simulink model "Microgrid_24h_Bhutan"  (Simulink 8.1)
settings: Solver=ode45  StartTime=0.0  StopTime=1  RelTol=1e-3
undefined symbols (not defined in the file or in its folder): Acid, Lead
libraries: powerlib x60, powerlib_extras x51, simulink x3, electricdrivelib x1
(part 2 of 2)

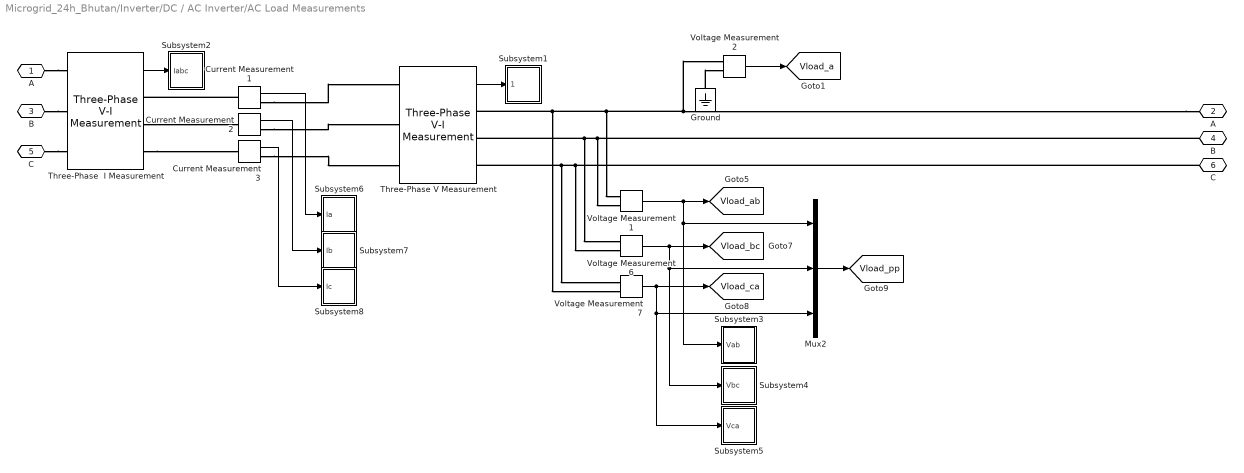
== system Microgrid_24h_Bhutan/Inverter/DC / AC Inverter/AC Load Measurements ==
  Current Measurement1 : powerlib/Measurements/Current Measurement  PhasorSimulation=off  OutputType=Complex  PSBequivalent=0
  Current Measurement2 : powerlib/Measurements/Current Measurement  PhasorSimulation=off  OutputType=Complex  PSBequivalent=0
  Current Measurement3 : powerlib/Measurements/Current Measurement  PhasorSimulation=off  OutputType=Complex  PSBequivalent=0
  Ground : powerlib/Elements/Ground  LConnTagsString=a
  Mux2 : Mux  Inputs=3
  Subsystem1 : Subsystem
  Subsystem2 : Subsystem
  Subsystem3 : Subsystem
  Subsystem4 : Subsystem
  Subsystem5 : Subsystem
  Subsystem6 : Subsystem
  Subsystem7 : Subsystem
  Subsystem8 : Subsystem
  Three-Phase V Measurement : powerlib/Measurements/Three-Phase V-I Measurement  VoltageMeasurement=phase-to-ground  SetLabelV=off  LabelV=Vabc  Vpu=off  VpuLL=off  CurrentMeasurement=no  SetLabelI=off  LabelI=Iabc  Ipu=off  Pbase=100e6  Vbase=500e3  OutputType=Complex  PhasorSimulation=off  PSBequivalent=0
  Three-Phase  I Measurement : powerlib/Measurements/Three-Phase V-I Measurement  VoltageMeasurement=no  SetLabelV=off  LabelV=Vabc  Vpu=off  VpuLL=off  CurrentMeasurement=yes  SetLabelI=off  LabelI=Iabc  Ipu=off  Pbase=100e6  Vbase=500e3  OutputType=Complex  PhasorSimulation=off  PSBequivalent=0
  Voltage Measurement{1..2,6..7} (4 alike) : powerlib/Measurements/Voltage Measurement  PhasorSimulation=off  OutputType=Complex  PSBequivalent=0
  A : PMIOPort  Port=1  Side=Left
  "A " : PMIOPort  Port=2  Side=Right
  B : PMIOPort  Port=3  Side=Left
  "B " : PMIOPort  Port=4  Side=Right
  C : PMIOPort  Port=5  Side=Left
  "C " : PMIOPort  Port=6  Side=Right
  tag scope: Vload_a=global, Vload_ab=global, Vload_bc=global, Vload_ca=global, Vload_pp=global
  wires:
  Three-Phase  I Measurement/1 -> Subsystem2/1(Iabc)
  Voltage Measurement1/1 -> [Vload_ab], Mux2/1, Subsystem3/1(Vab)
  Voltage Measurement6/1 -> [Vload_bc], Mux2/2, Subsystem4/1(Vbc)
  Voltage Measurement7/1 -> [Vload_ca], Mux2/3, Subsystem5/1(Vca)
  Mux2/1 -> [Vload_pp]
  Three-Phase V Measurement/1 -> Subsystem1/1(Vabc)
  Voltage Measurement2/1 -> [Vload_a]
  Current Measurement3/1 -> Subsystem8/1(Ic)
  Current Measurement2/1 -> Subsystem7/1(Ib)
  Current Measurement1/1 -> Subsystem6/1(Ia)
  connections:
  A/RConn1 -- Three-Phase  I Measurement/LConn1
  "A "/RConn1 -- Voltage Measurement1/LConn1 -- Three-Phase V Measurement/RConn1 -- Voltage Measurement7/LConn2 -- Voltage Measurement2/LConn1
  B/RConn1 -- Three-Phase  I Measurement/LConn2
  "B "/RConn1 -- Voltage Measurement1/LConn2 -- Three-Phase V Measurement/RConn2 -- Voltage Measurement6/LConn1
  C/RConn1 -- Three-Phase  I Measurement/LConn3
  "C "/RConn1 -- Voltage Measurement6/LConn2 -- Three-Phase V Measurement/RConn3 -- Voltage Measurement7/LConn1
  Ground/LConn1 -- Voltage Measurement2/LConn2
  Current Measurement1/LConn1 -- Three-Phase  I Measurement/RConn1
  Three-Phase  I Measurement/RConn2 -- Current Measurement2/LConn1
  Three-Phase  I Measurement/RConn3 -- Current Measurement3/LConn1
  Current Measurement3/RConn1 -- Three-Phase V Measurement/LConn3
  Current Measurement2/RConn1 -- Three-Phase V Measurement/LConn2
  Current Measurement1/RConn1 -- Three-Phase V Measurement/LConn1

== system Microgrid_24h_Bhutan/Inverter/DC BUS /Subsystem1 ==
  Idcinv : Inport
  LPF vq11 : powerlib_extras/Discrete  Control Blocks/Discrete 1st-Order Filter  FilterType=Lowpass  Tc=10e-3  Ts=5e-6  Initialize=off  Vac_Init=[0.8 -25 60]  Vdc_Init=0  PlotResponse=off  param1=[1 100 0.1]
  To Workspace1 : ToWorkspace  VariableName=Idcinv  SampleTime=-1
  To Workspace2 : ToWorkspace  VariableName=Idcinv1  SampleTime=-1
  tag scope: Idcinv=global
  wires:
  Idcinv/1 -> [Idcinv], To Workspace1/1, LPF vq11/1
  LPF vq11/1 -> To Workspace2/1

== system Microgrid_24h_Bhutan/Inverter/DC BUS /Subsystem2 ==
  Vdcinv : Inport
  LPF vq11 : powerlib_extras/Discrete  Control Blocks/Discrete 1st-Order Filter  FilterType=Lowpass  Tc=10e-3  Ts=5e-6  Initialize=off  Vac_Init=[0.8 -25 60]  Vdc_Init=0  PlotResponse=off  param1=[1 100 0.1]
  To Workspace1 : ToWorkspace  VariableName=Vdcinv  SampleTime=-1
  To Workspace2 : ToWorkspace  VariableName=Vdcinv1  SampleTime=-1
  tag scope: Vdcinv=global
  wires:
  Vdcinv/1 -> [Vdcinv], To Workspace1/1, LPF vq11/1
  LPF vq11/1 -> To Workspace2/1

== system Microgrid_24h_Bhutan/Inverter/Inverter Control/ Voltage Reference Generator ==
  Mux4 : Mux  Inputs=3
  Phase A reference : Sin  Amplitude=400*sqrt(2)/sqrt(3)  Frequency=2*pi*50  SampleTime=0
  Phase B reference : Sin  Amplitude=400*sqrt(2)/sqrt(3)  Frequency=2*pi*50  Phase=-2*pi/3  SampleTime=0
  Phase C reference : Sin  Amplitude=400*sqrt(2)/sqrt(3)  Frequency=2*pi*50  Phase=2*pi/3  SampleTime=0
  Product : Product  RndMeth=Zero
  Ramp : simulink/Sources/Ramp  slope=1/0.3  start=0  X0=0
  Saturation : Saturate  UpperLimit=1  LowerLimit=0
  Vabc* : Outport
  tag scope: Vabc_ref=global
  wires:
  Phase B reference/1 -> Mux4/2
  Phase A reference/1 -> Mux4/1
  Phase C reference/1 -> Mux4/3
  Ramp/1 -> Saturation/1
  Saturation/1 -> Product/2
  Mux4/1 -> Vabc*/1, [Vabc_ref]

== system Microgrid_24h_Bhutan/Inverter/Inverter Control/Cross Terms ==
  id* : Inport
  iq* : Inport  Port=2
  Gain1 : Gain  Gain=-2*pi*50*3e-3
  Gain2 : Gain  Gain=2*pi*50*3e-3
  " q" : Outport
  " d" : Outport  Port=2
  wires:
  id*/1 -> Gain1/1
  iq*/1 -> Gain2/1
  Gain1/1 -> " d"/1
  Gain2/1 -> " q"/1

== system Microgrid_24h_Bhutan/Inverter/Inverter Control/Current Ref. Generator ==
  note: evd
  note: evq
  evd : Inport
  evq : Inport  Port=2
  Divide : Product  Inputs=*/
  Divide1 : Product  Inputs=/*
  Scope24 : Scope
      settings: TimeRange=0.09  YMin=0.699626  YMax=0.699626  SaveName=ScopeData53
  Sum1 : Sum  Inputs=-+|
  Sum3 : Sum  Inputs=|++
  Zd : Gain  Gain=0.4559
  Zd1 : Gain  Gain=0.4559
  Zd^2+Zq^2 : Constant  Value=0.4559^2+0.1824^2
  Zq : Gain  Gain=0.1824
  Zq1 : Gain  Gain=0.1824
  id* : Outport
  iq* : Outport  Port=2
  tag scope: id_ref=global, iq_ref=global
  wires:
  Zd/1 -> Sum3/1
  Zq1/1 -> Sum3/2
  Zd1/1 -> Sum1/2
  Zq/1 -> Sum1/1
  Sum3/1 -> Divide/1
  Zd^2+Zq^2/1 -> Divide/2, Divide1/1, Scope24/1
  Sum1/1 -> Divide1/2
  evd/1 -> Zd/1, Zq/1
  evq/1 -> Zd1/1, Zq1/1
  Divide1/1 -> iq*/1, [iq_ref]
  Divide/1 -> id*/1, [id_ref]

== system Microgrid_24h_Bhutan/Inverter/Inverter Control/Frequency Reference Generator ==
  note: theta
  Constant : Constant  Value=2*pi
  Integrator : Integrator  ExternalReset=rising
  Relational Operator : RelationalOperator  OutDataTypeStr=boolean
  "f* " : Constant  Value=50
  w* : Gain  Gain=2*pi
  theta* : Outport
  tag scope: f_ref=global, theta=global
  wires:
  "f* "/1 -> w*/1, [f_ref]
  w*/1 -> Integrator/1
  Relational Operator/1 -> Integrator/2
  Constant/1 -> Relational Operator/2
  Integrator/1 -> Relational Operator/1, theta*/1, [theta]

== system Microgrid_24h_Bhutan/Inverter/Inverter Control/Iabc  - idq ==
  Iabc : Inport
  theta : Inport  Port=2
  Demux : Demux  Outputs=2
  abc  - alfa/beta : Subsystem
  alfa/beta - dq : Subsystem
  iq : Outport
  id : Outport  Port=2
  tag scope: id=global, iq=global
  wires:
  theta/1 -> alfa/beta - dq/2(theta)
  Iabc/1 -> abc  - alfa/beta/1(abc)
  abc  - alfa/beta/1(alfa/beta) -> alfa/beta - dq/1(alfa/beta)
  alfa/beta - dq/1(d/q) -> Demux/1
  Demux/1 -> id/1, [id]
  Demux/2 -> iq/1, [iq]

== system Microgrid_24h_Bhutan/Inverter/Inverter Control/Iabc  - idq1 ==
  Iabc : Inport
  theta : Inport  Port=2
  Demux : Demux  Outputs=2
  abc  - alfa/beta : Subsystem
  alfa/beta - dq : Subsystem
  iq : Outport
  id : Outport  Port=2
  tag scope: id2=global, iq2=global
  wires:
  Demux/2 -> [iq2], iq/1
  Demux/1 -> [id2], id/1
  alfa/beta - dq/1(d/q) -> Demux/1
  abc  - alfa/beta/1(alfa/beta) -> alfa/beta - dq/1(alfa/beta)
  Iabc/1 -> abc  - alfa/beta/1(abc)
  theta/1 -> alfa/beta - dq/2(theta)

== system Microgrid_24h_Bhutan/Inverter/Inverter Control/Iabc  - idq2 ==
  Iabc : Inport
  theta : Inport  Port=2
  Demux : Demux  Outputs=2
  abc  - alfa/beta : Subsystem
  alfa/beta - dq : Subsystem
  iq : Outport
  id : Outport  Port=2
  tag scope: id3=global, iq3=global
  wires:
  theta/1 -> alfa/beta - dq/2(theta)
  Iabc/1 -> abc  - alfa/beta/1(abc)
  abc  - alfa/beta/1(alfa/beta) -> alfa/beta - dq/1(alfa/beta)
  alfa/beta - dq/1(d/q) -> Demux/1
  Demux/1 -> id/1, [id3]
  Demux/2 -> iq/1, [iq3]

== system Microgrid_24h_Bhutan/Inverter/Inverter Control/PI id ==
  e : Inport
  Gain1 : Gain  Gain=50
  Gain2 : Gain  Gain=500
  Integrator : Integrator
  Saturation : Saturate  UpperLimit=inf  LowerLimit=-inf
  Sum1 : Sum  Inputs=|++
  " " : Outport
  wires:
  Sum1/1 -> Saturation/1
  Integrator/1 -> Sum1/2
  Gain1/1 -> Sum1/1
  e/1 -> Gain2/1, Gain1/1
  Gain2/1 -> Integrator/1
  Saturation/1 -> " "/1

== system Microgrid_24h_Bhutan/Inverter/Inverter Control/PI iq ==
  e : Inport
  Gain1 : Gain  Gain=50
  Gain2 : Gain  Gain=500
  Integrator : Integrator
  Saturation : Saturate  UpperLimit=inf  LowerLimit=-inf
  Sum1 : Sum  Inputs=|++
  " " : Outport
  wires:
  Saturation/1 -> " "/1
  Gain2/1 -> Integrator/1
  e/1 -> Gain1/1, Gain2/1
  Gain1/1 -> Sum1/1
  Integrator/1 -> Sum1/2
  Sum1/1 -> Saturation/1

== system Microgrid_24h_Bhutan/Inverter/Inverter Control/PI vd ==
  e : Inport
  Gain1 : Gain  Gain=2
  Gain2 : Gain  Gain=20
  Integrator : Integrator
  Saturation : Saturate  UpperLimit=inf  LowerLimit=-inf
  Sum1 : Sum  Inputs=|++
  " " : Outport
  wires:
  Saturation/1 -> " "/1
  Gain2/1 -> Integrator/1
  e/1 -> Gain1/1, Gain2/1
  Gain1/1 -> Sum1/1
  Integrator/1 -> Sum1/2
  Sum1/1 -> Saturation/1

== system Microgrid_24h_Bhutan/Inverter/Inverter Control/PI vq ==
  e : Inport
  Gain1 : Gain  Gain=2
  Gain2 : Gain  Gain=2
  Integrator : Integrator
  Saturation : Saturate  UpperLimit=inf  LowerLimit=-inf
  Sum1 : Sum  Inputs=|++
  " " : Outport
  wires:
  Sum1/1 -> Saturation/1
  Integrator/1 -> Sum1/2
  Gain1/1 -> Sum1/1
  e/1 -> Gain2/1, Gain1/1
  Gain2/1 -> Integrator/1
  Saturation/1 -> " "/1

== system Microgrid_24h_Bhutan/Inverter/Inverter Control/PWM ==
  Uabc_ref : Inport
  Gain2 : Gain  Gain=2/1000
  PWM Generator : powerlib_extras/Control  Blocks/PWM Generator  GeneratorMode="3-arm  bridge (6 pulses)"  Fc=10000  Internal=off  mIndex=0.4  Freq=60  Phase=0
  S : Outport
  tag scope: m_index=global, pulses=global
  wires:
  PWM Generator/1 -> S/1, [pulses]
  Uabc_ref/1 -> Gain2/1
  Gain2/1 -> PWM Generator/1, [m_index]

== system Microgrid_24h_Bhutan/Inverter/Inverter Control/Vabc  - vdq ==
  Vabc : Inport
  theta : Inport  Port=2
  Demux : Demux  Outputs=2
  abc  - alfa/beta : Subsystem
  alfa/beta - dq : Subsystem
  vq : Outport
  vd : Outport  Port=2
  tag scope: vd=global, vq=global
  wires:
  Demux/2 -> vq/1, [vq]
  Demux/1 -> vd/1, [vd]
  alfa/beta - dq/1(d/q) -> Demux/1
  abc  - alfa/beta/1(alfa/beta) -> alfa/beta - dq/1(alfa/beta)
  Vabc/1 -> abc  - alfa/beta/1(abc)
  theta/1 -> alfa/beta - dq/2(theta)

== system Microgrid_24h_Bhutan/Inverter/Inverter Control/Vabc  - vdq1 ==
  Vabc : Inport
  theta : Inport  Port=2
  Demux : Demux  Outputs=2
  abc  - alfa/beta : Subsystem
  alfa/beta - dq : Subsystem
  vq : Outport
  vd : Outport  Port=2
  tag scope: vd2=global, vq2=global
  wires:
  theta/1 -> alfa/beta - dq/2(theta)
  Vabc/1 -> abc  - alfa/beta/1(abc)
  abc  - alfa/beta/1(alfa/beta) -> alfa/beta - dq/1(alfa/beta)
  alfa/beta - dq/1(d/q) -> Demux/1
  Demux/1 -> [vd2], vd/1
  Demux/2 -> [vq2], vq/1

== system Microgrid_24h_Bhutan/Inverter/Inverter Control/Vabc  - vdq2 ==
  Vabc : Inport
  theta : Inport  Port=2
  Demux : Demux  Outputs=2
  abc  - alfa/beta : Subsystem
  alfa/beta - dq : Subsystem
  vq : Outport
  vd : Outport  Port=2
  tag scope: vd3=global, vq3=global
  wires:
  Demux/2 -> vq/1, [vq3]
  Demux/1 -> vd/1, [vd3]
  alfa/beta - dq/1(d/q) -> Demux/1
  abc  - alfa/beta/1(alfa/beta) -> alfa/beta - dq/1(alfa/beta)
  Vabc/1 -> abc  - alfa/beta/1(abc)
  theta/1 -> alfa/beta - dq/2(theta)

== system Microgrid_24h_Bhutan/Inverter/Inverter Control/Vabc*  - vdq* ==
  Vabc* : Inport
  theta : Inport  Port=2
  Demux : Demux  Outputs=2
  abc  - alfa/beta : Subsystem
  alfa/beta - dq : Subsystem
  vd* : Outport
  vq* : Outport  Port=2
  tag scope: vd_ref=global, vq_ref=global
  wires:
  theta/1 -> alfa/beta - dq/2(theta)
  Vabc*/1 -> abc  - alfa/beta/1(abc)
  abc  - alfa/beta/1(alfa/beta) -> alfa/beta - dq/1(alfa/beta)
  alfa/beta - dq/1(d/q) -> Demux/1
  Demux/1 -> vd*/1, [vd_ref]
  Demux/2 -> vq*/1, [vq_ref]

== system Microgrid_24h_Bhutan/Inverter/Inverter Control/vdq - Vabc ==
  Ud/Uq : Inport
  theta : Inport  Port=2
  alfa/beta - abc : Subsystem
  d/q - alfa/beta : Subsystem
  Uabc_ref : Outport
  wires:
  d/q - alfa/beta/1(alfa/beta) -> alfa/beta - abc/1(alfa/beta)
  Ud/Uq/1 -> d/q - alfa/beta/1(d/q)
  alfa/beta - abc/1(abc) -> Uabc_ref/1
  theta/1 -> d/q - alfa/beta/2(tita)

== system Microgrid_24h_Bhutan/Subsystem/Inverter Control  Measurements/Subsystem1 ==
  vd_ref : Inport
  To Workspace1 : ToWorkspace  VariableName=vd_ref  SampleTime=-1
  Zero-Order Hold1 : ZeroOrderHold  SampleTime=5e-6
  wires:
  vd_ref/1 -> Zero-Order Hold1/1
  Zero-Order Hold1/1 -> To Workspace1/1

== system Microgrid_24h_Bhutan/Subsystem/Inverter Control  Measurements/Subsystem10 ==
  f_ref : Inport
  To Workspace1 : ToWorkspace  VariableName=f_ref  SampleTime=-1
  Zero-Order Hold1 : ZeroOrderHold  SampleTime=5e-6
  wires:
  f_ref/1 -> Zero-Order Hold1/1
  Zero-Order Hold1/1 -> To Workspace1/1

== system Microgrid_24h_Bhutan/Subsystem/Inverter Control  Measurements/Subsystem11 ==
  theta : Inport
  To Workspace1 : ToWorkspace  VariableName=theta  SampleTime=-1
  Zero-Order Hold1 : ZeroOrderHold  SampleTime=5e-6
  wires:
  theta/1 -> Zero-Order Hold1/1
  Zero-Order Hold1/1 -> To Workspace1/1

== system Microgrid_24h_Bhutan/Subsystem/Inverter Control  Measurements/Subsystem12 ==
  m_index : Inport
  To Workspace1 : ToWorkspace  VariableName=m_index  SampleTime=-1
  Zero-Order Hold1 : ZeroOrderHold  SampleTime=5e-6
  wires:
  m_index/1 -> Zero-Order Hold1/1
  Zero-Order Hold1/1 -> To Workspace1/1

== system Microgrid_24h_Bhutan/Subsystem/Inverter Control  Measurements/Subsystem13 ==
  pulses : Inport
  To Workspace1 : ToWorkspace  VariableName=pulses  SampleTime=-1
  Zero-Order Hold1 : ZeroOrderHold  SampleTime=5e-6
  wires:
  pulses/1 -> Zero-Order Hold1/1
  Zero-Order Hold1/1 -> To Workspace1/1

== system Microgrid_24h_Bhutan/Subsystem/Inverter Control  Measurements/Subsystem2 ==
  vq_ref : Inport
  To Workspace1 : ToWorkspace  VariableName=vq_ref  SampleTime=-1
  Zero-Order Hold1 : ZeroOrderHold  SampleTime=5e-6
  wires:
  vq_ref/1 -> Zero-Order Hold1/1
  Zero-Order Hold1/1 -> To Workspace1/1

== system Microgrid_24h_Bhutan/Subsystem/Inverter Control  Measurements/Subsystem3 ==
  vd : Inport
  To Workspace1 : ToWorkspace  VariableName=vd  SampleTime=-1
  Zero-Order Hold1 : ZeroOrderHold  SampleTime=5e-6
  wires:
  vd/1 -> Zero-Order Hold1/1
  Zero-Order Hold1/1 -> To Workspace1/1

== system Microgrid_24h_Bhutan/Subsystem/Inverter Control  Measurements/Subsystem4 ==
  vq : Inport
  To Workspace1 : ToWorkspace  VariableName=vq  SampleTime=-1
  Zero-Order Hold1 : ZeroOrderHold  SampleTime=5e-6
  wires:
  vq/1 -> Zero-Order Hold1/1
  Zero-Order Hold1/1 -> To Workspace1/1

== system Microgrid_24h_Bhutan/Subsystem/Inverter Control  Measurements/Subsystem5 ==
  id_ref : Inport
  To Workspace1 : ToWorkspace  VariableName=id_ref  SampleTime=-1
  Zero-Order Hold1 : ZeroOrderHold  SampleTime=5e-6
  wires:
  id_ref/1 -> Zero-Order Hold1/1
  Zero-Order Hold1/1 -> To Workspace1/1

== system Microgrid_24h_Bhutan/Subsystem/Inverter Control  Measurements/Subsystem6 ==
  id : Inport
  To Workspace1 : ToWorkspace  VariableName=id  SampleTime=-1
  Zero-Order Hold1 : ZeroOrderHold  SampleTime=5e-6
  wires:
  id/1 -> Zero-Order Hold1/1
  Zero-Order Hold1/1 -> To Workspace1/1

== system Microgrid_24h_Bhutan/Subsystem/Inverter Control  Measurements/Subsystem7 ==
  iq_ref : Inport
  To Workspace1 : ToWorkspace  VariableName=iq_ref  SampleTime=-1
  Zero-Order Hold1 : ZeroOrderHold  SampleTime=5e-6
  wires:
  iq_ref/1 -> Zero-Order Hold1/1
  Zero-Order Hold1/1 -> To Workspace1/1

== system Microgrid_24h_Bhutan/Subsystem/Inverter Control  Measurements/Subsystem8 ==
  iq : Inport
  To Workspace1 : ToWorkspace  VariableName=iq  SampleTime=-1
  Zero-Order Hold1 : ZeroOrderHold  SampleTime=5e-6
  wires:
  iq/1 -> Zero-Order Hold1/1
  Zero-Order Hold1/1 -> To Workspace1/1

== system Microgrid_24h_Bhutan/Subsystem/Inverter Control  Measurements/Subsystem9 ==
  Vabc_ref : Inport
  To Workspace1 : ToWorkspace  VariableName=Vabc_ref  SampleTime=-1
  Zero-Order Hold1 : ZeroOrderHold  SampleTime=5e-6
  wires:
  Vabc_ref/1 -> Zero-Order Hold1/1
  Zero-Order Hold1/1 -> To Workspace1/1

== system Microgrid_24h_Bhutan/Subsystem/Inverter Control  Measurements3/PLL ==
  Vabc : Inport
  Demux : Demux  Outputs=2
  Integrator : Integrator
  PI : Subsystem
  Subsystem3 : Subsystem
  Terminator : Terminator
  abc  - d/q : Subsystem
  wires:
  Vabc/1 -> abc  - d/q/1(abc)
  Integrator/1 -> abc  - d/q/2(tita)
  PI/1(w) -> Integrator/1, Subsystem3/1(wabc)
  Demux/2 -> PI/1(e)
  abc  - d/q/1(d/q) -> Demux/1
  Demux/1 -> Terminator/1

== system Microgrid_24h_Bhutan/Subsystem/Inverter Control  Measurements3/Subsystem ==
  LPF vq2 : powerlib_extras/Discrete  Control Blocks/Discrete 1st-Order Filter  FilterType=Lowpass  Tc=10e-3  Ts=5e-6  Initialize=off  Vac_Init=[0.8 -25 60]  Vdc_Init=0  PlotResponse=off  param1=[1 100 0.1]
  LPF vq3 : powerlib_extras/Discrete  Control Blocks/Discrete 1st-Order Filter  FilterType=Lowpass  Tc=10e-3  Ts=5e-6  Initialize=off  Vac_Init=[0.8 -25 60]  Vdc_Init=0  PlotResponse=off  param1=[1 100 0.1]
  LPF vq4 : powerlib_extras/Discrete  Control Blocks/Discrete 1st-Order Filter  FilterType=Lowpass  Tc=10e-3  Ts=5e-6  Initialize=off  Vac_Init=[0.8 -25 60]  Vdc_Init=0  PlotResponse=off  param1=[1 100 0.1]
  Mux : Mux  Inputs=3
  Vabc : Outport
  wires:
  [Vab] -> LPF vq2/1
  [Vbc] -> LPF vq3/1
  [Vca] -> LPF vq4/1
  LPF vq2/1 -> Mux/1
  LPF vq3/1 -> Mux/2
  LPF vq4/1 -> Mux/3
  Mux/1 -> Vabc/1

== system Microgrid_24h_Bhutan/Subsystem/Load Power Calculation/Subsystem1 ==
  Qacload : Inport
  LPF vq7 : powerlib_extras/Discrete  Control Blocks/Discrete 1st-Order Filter  FilterType=Lowpass  Tc=10e-3  Ts=5e-6  Initialize=off  Vac_Init=[0.8 -25 60]  Vdc_Init=0  PlotResponse=off  param1=[1 100 0.1]
  To Workspace1 : ToWorkspace  VariableName=Qacload  SampleTime=-1
  To Workspace2 : ToWorkspace  VariableName=Qacload1  SampleTime=-1
  Zero-Order Hold : ZeroOrderHold  SampleTime=5e-6
  tag scope: Qacload=global
  wires:
  Qacload/1 -> Zero-Order Hold/1
  Zero-Order Hold/1 -> [Qacload], To Workspace2/1, LPF vq7/1
  LPF vq7/1 -> To Workspace1/1

== system Microgrid_24h_Bhutan/Subsystem/Load Power Calculation/Subsystem2 ==
  Pload : Inport
  LPF vq7 : powerlib_extras/Discrete  Control Blocks/Discrete 1st-Order Filter  FilterType=Lowpass  Tc=10e-3  Ts=5e-6  Initialize=off  Vac_Init=[0.8 -25 60]  Vdc_Init=0  PlotResponse=off  param1=[1 100 0.1]
  To Workspace1 : ToWorkspace  VariableName=Pacload  SampleTime=-1
  To Workspace2 : ToWorkspace  VariableName=Pacload1  SampleTime=-1
  Zero-Order Hold : ZeroOrderHold  SampleTime=5e-6
  tag scope: Pacload=global
  wires:
  Pload/1 -> Zero-Order Hold/1
  Zero-Order Hold/1 -> [Pacload], To Workspace2/1, LPF vq7/1
  LPF vq7/1 -> To Workspace1/1

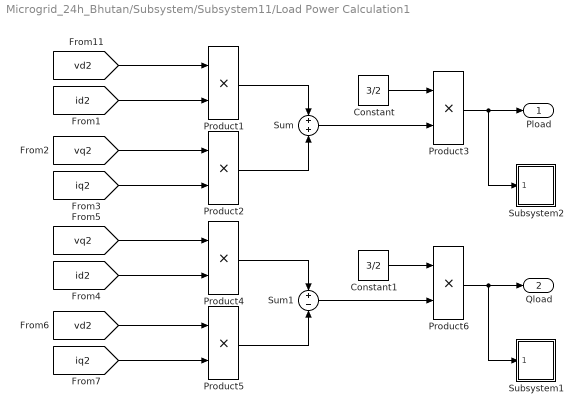
== system Microgrid_24h_Bhutan/Subsystem/Subsystem11/Load Power Calculation1 ==
  Constant : Constant  Value=3/2
  Constant1 : Constant  Value=3/2
  Product{1..6} (6 alike) : Product  RndMeth=Zero
  Subsystem1 : Subsystem
  Subsystem2 : Subsystem
  Sum : Sum  Inputs=+|+
  Sum1 : Sum  Inputs=+|-
  Pload : Outport
  Qload : Outport  Port=2
  wires:
  Product6/1 -> Qload/1, Subsystem1/1(Qacload)
  Constant1/1 -> Product6/1
  Sum1/1 -> Product6/2
  Product5/1 -> Sum1/2
  Product4/1 -> Sum1/1
  [iq2] -> Product5/2
  [vd2] -> Product5/1
  [id2] -> Product4/2
  [vq2] -> Product4/1
  Product3/1 -> Pload/1, Subsystem2/1(Pload)
  Constant/1 -> Product3/1
  Sum/1 -> Product3/2
  Product2/1 -> Sum/2
  Product1/1 -> Sum/1
  [iq2] -> Product2/2
  [vq2] -> Product2/1
  [id2] -> Product1/2
  [vd2] -> Product1/1

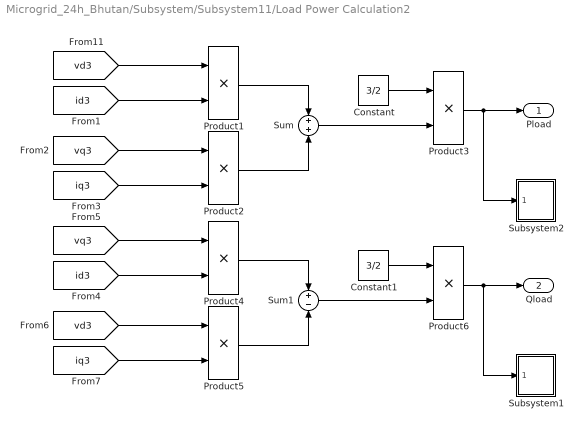
== system Microgrid_24h_Bhutan/Subsystem/Subsystem11/Load Power Calculation2 ==
  Constant : Constant  Value=3/2
  Constant1 : Constant  Value=3/2
  Product{1..6} (6 alike) : Product  RndMeth=Zero
  Subsystem1 : Subsystem
  Subsystem2 : Subsystem
  Sum : Sum  Inputs=+|+
  Sum1 : Sum  Inputs=+|-
  Pload : Outport
  Qload : Outport  Port=2
  wires:
  [vd3] -> Product1/1
  [id3] -> Product1/2
  [vq3] -> Product2/1
  [iq3] -> Product2/2
  Product1/1 -> Sum/1
  Product2/1 -> Sum/2
  Sum/1 -> Product3/2
  Constant/1 -> Product3/1
  Product3/1 -> Pload/1, Subsystem2/1(Pload)
  [vq3] -> Product4/1
  [id3] -> Product4/2
  [vd3] -> Product5/1
  [iq3] -> Product5/2
  Product4/1 -> Sum1/1
  Product5/1 -> Sum1/2
  Sum1/1 -> Product6/2
  Constant1/1 -> Product6/1
  Product6/1 -> Qload/1, Subsystem1/1(Qacload)

== system Microgrid_24h_Bhutan/Inverter/DC / AC Inverter/AC Load Measurements/Subsystem1 ==
  Vabc : Inport
  To Workspace1 : ToWorkspace  VariableName=Vabc  SampleTime=-1
  tag scope: Vabc=global
  wires:
  Vabc/1 -> To Workspace1/1, [Vabc]

== system Microgrid_24h_Bhutan/Inverter/DC / AC Inverter/AC Load Measurements/Subsystem2 ==
  Iabc : Inport
  To Workspace1 : ToWorkspace  VariableName=Iabc  SampleTime=-1
  tag scope: Iabc=global
  wires:
  Iabc/1 -> [Iabc], To Workspace1/1

== system Microgrid_24h_Bhutan/Inverter/DC / AC Inverter/AC Load Measurements/Subsystem3 ==
  Vab : Inport
  To Workspace1 : ToWorkspace  VariableName=Vab  SampleTime=-1
  To Workspace2 : ToWorkspace  VariableName=Vab_s  SampleTime=-1  SaveFormat=Structure
  To Workspace3 : ToWorkspace  VariableName=Vab_st  SampleTime=-1  SaveFormat=Structure With Time
  tag scope: Vab=global
  wires:
  Vab/1 -> [Vab], To Workspace1/1, To Workspace2/1, To Workspace3/1

== system Microgrid_24h_Bhutan/Inverter/DC / AC Inverter/AC Load Measurements/Subsystem4 ==
  Vbc : Inport
  To Workspace1 : ToWorkspace  VariableName=Vbc  SampleTime=-1
  tag scope: Vbc=global
  wires:
  Vbc/1 -> To Workspace1/1, [Vbc]

== system Microgrid_24h_Bhutan/Inverter/DC / AC Inverter/AC Load Measurements/Subsystem5 ==
  Vca : Inport
  To Workspace1 : ToWorkspace  VariableName=Vca  SampleTime=-1
  tag scope: Vca=global
  wires:
  Vca/1 -> [Vca], To Workspace1/1

== system Microgrid_24h_Bhutan/Inverter/DC / AC Inverter/AC Load Measurements/Subsystem6 ==
  Ia : Inport
  To Workspace1 : ToWorkspace  VariableName=Ia  SampleTime=-1
  tag scope: Ia=global
  wires:
  Ia/1 -> To Workspace1/1, [Ia]

== system Microgrid_24h_Bhutan/Inverter/DC / AC Inverter/AC Load Measurements/Subsystem7 ==
  Ib : Inport
  To Workspace1 : ToWorkspace  VariableName=Ib  SampleTime=-1
  tag scope: Ib=global
  wires:
  Ib/1 -> [Ib], To Workspace1/1

== system Microgrid_24h_Bhutan/Inverter/DC / AC Inverter/AC Load Measurements/Subsystem8 ==
  Ic : Inport
  To Workspace1 : ToWorkspace  VariableName=Ic  SampleTime=-1
  tag scope: Ic=global
  wires:
  Ic/1 -> To Workspace1/1, [Ic]

== system Microgrid_24h_Bhutan/Inverter/Inverter Control/Iabc  - idq/abc  - alfa/beta ==
  abc : Inport
  Mux : Mux  Inputs=2
  d_s : Fcn  Expr=(-1/sqrt(3)*u(2))+(1/sqrt(3)*u(3))
  q_s : Fcn  Expr=(2/3)*u(1)-(1/3)*u(2)-(1/3)*u(3)
  alfa/beta : Outport
  wires:
  abc/1 -> q_s/1, d_s/1
  d_s/1 -> Mux/1
  q_s/1 -> Mux/2
  Mux/1 -> alfa/beta/1

== system Microgrid_24h_Bhutan/Inverter/Inverter Control/Iabc  - idq/alfa/beta - dq ==
  alfa/beta : Inport
  theta : Inport  Port=2
  Mux : Mux  Inputs=2
  Mux1 : Mux  Inputs=2
  d : Fcn  Expr=u(2)*sin(u(3)) + u(1)*cos(u(3))
  q : Fcn  Expr=-u(1)*sin(u(3)) + u(2)*cos(u(3))
  d/q : Outport
  wires:
  d/1 -> Mux/1
  q/1 -> Mux/2
  Mux/1 -> d/q/1
  alfa/beta/1 -> Mux1/1
  theta/1 -> Mux1/2
  Mux1/1 -> d/1, q/1

== system Microgrid_24h_Bhutan/Inverter/Inverter Control/Iabc  - idq1/abc  - alfa/beta ==
  abc : Inport
  Mux : Mux  Inputs=2
  d_s : Fcn  Expr=(-1/sqrt(3)*u(2))+(1/sqrt(3)*u(3))
  q_s : Fcn  Expr=(2/3)*u(1)-(1/3)*u(2)-(1/3)*u(3)
  alfa/beta : Outport
  wires:
  Mux/1 -> alfa/beta/1
  q_s/1 -> Mux/2
  d_s/1 -> Mux/1
  abc/1 -> d_s/1, q_s/1

== system Microgrid_24h_Bhutan/Inverter/Inverter Control/Iabc  - idq1/alfa/beta - dq ==
  alfa/beta : Inport
  theta : Inport  Port=2
  Mux : Mux  Inputs=2
  Mux1 : Mux  Inputs=2
  d : Fcn  Expr=u(2)*sin(u(3)) + u(1)*cos(u(3))
  q : Fcn  Expr=-u(1)*sin(u(3)) + u(2)*cos(u(3))
  d/q : Outport
  wires:
  Mux1/1 -> q/1, d/1
  theta/1 -> Mux1/2
  alfa/beta/1 -> Mux1/1
  Mux/1 -> d/q/1
  q/1 -> Mux/2
  d/1 -> Mux/1

== system Microgrid_24h_Bhutan/Inverter/Inverter Control/Iabc  - idq2/abc  - alfa/beta ==
  abc : Inport
  Mux : Mux  Inputs=2
  d_s : Fcn  Expr=(-1/sqrt(3)*u(2))+(1/sqrt(3)*u(3))
  q_s : Fcn  Expr=(2/3)*u(1)-(1/3)*u(2)-(1/3)*u(3)
  alfa/beta : Outport
  wires:
  abc/1 -> q_s/1, d_s/1
  d_s/1 -> Mux/1
  q_s/1 -> Mux/2
  Mux/1 -> alfa/beta/1

== system Microgrid_24h_Bhutan/Inverter/Inverter Control/Iabc  - idq2/alfa/beta - dq ==
  alfa/beta : Inport
  theta : Inport  Port=2
  Mux : Mux  Inputs=2
  Mux1 : Mux  Inputs=2
  d : Fcn  Expr=u(2)*sin(u(3)) + u(1)*cos(u(3))
  q : Fcn  Expr=-u(1)*sin(u(3)) + u(2)*cos(u(3))
  d/q : Outport
  wires:
  d/1 -> Mux/1
  q/1 -> Mux/2
  Mux/1 -> d/q/1
  alfa/beta/1 -> Mux1/1
  theta/1 -> Mux1/2
  Mux1/1 -> d/1, q/1

== system Microgrid_24h_Bhutan/Inverter/Inverter Control/Vabc  - vdq/abc  - alfa/beta ==
  abc : Inport
  Mux : Mux  Inputs=2
  d_s : Fcn  Expr=(-1/sqrt(3)*u(2))+(1/sqrt(3)*u(3))
  q_s : Fcn  Expr=(2/3)*u(1)-(1/3)*u(2)-(1/3)*u(3)
  alfa/beta : Outport
  wires:
  Mux/1 -> alfa/beta/1
  q_s/1 -> Mux/2
  d_s/1 -> Mux/1
  abc/1 -> d_s/1, q_s/1

== system Microgrid_24h_Bhutan/Inverter/Inverter Control/Vabc  - vdq/alfa/beta - dq ==
  alfa/beta : Inport
  theta : Inport  Port=2
  Mux : Mux  Inputs=2
  Mux1 : Mux  Inputs=2
  d : Fcn  Expr=u(2)*sin(u(3)) + u(1)*cos(u(3))
  q : Fcn  Expr=-u(1)*sin(u(3)) + u(2)*cos(u(3))
  d/q : Outport
  wires:
  Mux1/1 -> q/1, d/1
  theta/1 -> Mux1/2
  alfa/beta/1 -> Mux1/1
  Mux/1 -> d/q/1
  q/1 -> Mux/2
  d/1 -> Mux/1

== system Microgrid_24h_Bhutan/Inverter/Inverter Control/Vabc  - vdq1/abc  - alfa/beta ==
  abc : Inport
  Mux : Mux  Inputs=2
  d_s : Fcn  Expr=(-1/sqrt(3)*u(2))+(1/sqrt(3)*u(3))
  q_s : Fcn  Expr=(2/3)*u(1)-(1/3)*u(2)-(1/3)*u(3)
  alfa/beta : Outport
  wires:
  abc/1 -> q_s/1, d_s/1
  d_s/1 -> Mux/1
  q_s/1 -> Mux/2
  Mux/1 -> alfa/beta/1

== system Microgrid_24h_Bhutan/Inverter/Inverter Control/Vabc  - vdq1/alfa/beta - dq ==
  alfa/beta : Inport
  theta : Inport  Port=2
  Mux : Mux  Inputs=2
  Mux1 : Mux  Inputs=2
  d : Fcn  Expr=u(2)*sin(u(3)) + u(1)*cos(u(3))
  q : Fcn  Expr=-u(1)*sin(u(3)) + u(2)*cos(u(3))
  d/q : Outport
  wires:
  d/1 -> Mux/1
  q/1 -> Mux/2
  Mux/1 -> d/q/1
  alfa/beta/1 -> Mux1/1
  theta/1 -> Mux1/2
  Mux1/1 -> d/1, q/1

== system Microgrid_24h_Bhutan/Inverter/Inverter Control/Vabc  - vdq2/abc  - alfa/beta ==
  abc : Inport
  Mux : Mux  Inputs=2
  d_s : Fcn  Expr=(-1/sqrt(3)*u(2))+(1/sqrt(3)*u(3))
  q_s : Fcn  Expr=(2/3)*u(1)-(1/3)*u(2)-(1/3)*u(3)
  alfa/beta : Outport
  wires:
  Mux/1 -> alfa/beta/1
  q_s/1 -> Mux/2
  d_s/1 -> Mux/1
  abc/1 -> d_s/1, q_s/1

== system Microgrid_24h_Bhutan/Inverter/Inverter Control/Vabc  - vdq2/alfa/beta - dq ==
  alfa/beta : Inport
  theta : Inport  Port=2
  Mux : Mux  Inputs=2
  Mux1 : Mux  Inputs=2
  d : Fcn  Expr=u(2)*sin(u(3)) + u(1)*cos(u(3))
  q : Fcn  Expr=-u(1)*sin(u(3)) + u(2)*cos(u(3))
  d/q : Outport
  wires:
  Mux1/1 -> q/1, d/1
  theta/1 -> Mux1/2
  alfa/beta/1 -> Mux1/1
  Mux/1 -> d/q/1
  q/1 -> Mux/2
  d/1 -> Mux/1

== system Microgrid_24h_Bhutan/Inverter/Inverter Control/Vabc*  - vdq*/abc  - alfa/beta ==
  abc : Inport
  Mux : Mux  Inputs=2
  d_s : Fcn  Expr=(-1/sqrt(3)*u(2))+(1/sqrt(3)*u(3))
  q_s : Fcn  Expr=(2/3)*u(1)-(1/3)*u(2)-(1/3)*u(3)
  alfa/beta : Outport
  wires:
  abc/1 -> q_s/1, d_s/1
  d_s/1 -> Mux/1
  q_s/1 -> Mux/2
  Mux/1 -> alfa/beta/1

== system Microgrid_24h_Bhutan/Inverter/Inverter Control/Vabc*  - vdq*/alfa/beta - dq ==
  alfa/beta : Inport
  theta : Inport  Port=2
  Mux : Mux  Inputs=2
  Mux1 : Mux  Inputs=2
  d : Fcn  Expr=u(2)*sin(u(3)) + u(1)*cos(u(3))
  q : Fcn  Expr=-u(1)*sin(u(3)) + u(2)*cos(u(3))
  d/q : Outport
  wires:
  d/1 -> Mux/1
  q/1 -> Mux/2
  Mux/1 -> d/q/1
  alfa/beta/1 -> Mux1/1
  theta/1 -> Mux1/2
  Mux1/1 -> d/1, q/1

== system Microgrid_24h_Bhutan/Inverter/Inverter Control/vdq - Vabc/alfa/beta - abc ==
  alfa/beta : Inport
  Mux : Mux  Inputs=3
  a : Fcn  Expr=u[2]
  b : Fcn  Expr=-sqrt(3)/2*u[1]-0.5*u[2]
  c : Fcn  Expr=sqrt(3)/2*u[1]-0.5*u[2]
  abc : Outport
  tag scope: Vca_ref=global, Vcb_ref=global, Vcc_ref=global
  wires:
  alfa/beta/1 -> c/1, a/1, b/1
  Mux/1 -> abc/1
  c/1 -> Mux/3, [Vcc_ref]
  b/1 -> Mux/2, [Vcb_ref]
  a/1 -> Mux/1, [Vca_ref]

== system Microgrid_24h_Bhutan/Inverter/Inverter Control/vdq - Vabc/d/q - alfa/beta ==
  d/q : Inport
  tita : Inport  Port=2
  Mux : Mux  Inputs=2
  Mux1 : Mux  Inputs=2
  a : Fcn  Expr=-u[2]*sin(u[3]) + u[1]*cos(u[3])
  b : Fcn  Expr=u[1]*sin(u[3]) + u[2]*cos(u[3])
  alfa/beta : Outport
  wires:
  Mux1/1 -> b/1, a/1
  tita/1 -> Mux1/2
  d/q/1 -> Mux1/1
  a/1 -> Mux/1
  b/1 -> Mux/2
  Mux/1 -> alfa/beta/1

== system Microgrid_24h_Bhutan/Subsystem/Inverter Control  Measurements3/PLL/PI ==
  e : Inport
  Gain1 : Gain  Gain=10
  Gain2 : Gain  Gain=100
  Integrator : Integrator
  Saturation : Saturate  UpperLimit=inf  LowerLimit=-inf
  Sum1 : Sum  Inputs=|++
  w : Outport
  wires:
  Integrator/1 -> Sum1/2
  Gain1/1 -> Sum1/1
  e/1 -> Gain2/1, Gain1/1
  Gain2/1 -> Integrator/1
  Saturation/1 -> w/1
  Sum1/1 -> Saturation/1

== system Microgrid_24h_Bhutan/Subsystem/Inverter Control  Measurements3/PLL/Subsystem3 ==
  wabc : Inport
  LPF vq7 : powerlib_extras/Discrete  Control Blocks/Discrete 1st-Order Filter  FilterType=Lowpass  Tc=10e-3  Ts=5e-6  Initialize=off  Vac_Init=[0.8 -25 60]  Vdc_Init=0  PlotResponse=off  param1=[1 100 0.1]
  To Workspace1 : ToWorkspace  VariableName=wabc_real  SampleTime=-1
  To Workspace2 : ToWorkspace  VariableName=wabc_real_fil  SampleTime=-1
  Zero-Order Hold : ZeroOrderHold  SampleTime=5e-6
  tag scope: w_abc=global
  wires:
  LPF vq7/1 -> To Workspace2/1
  wabc/1 -> Zero-Order Hold/1
  Zero-Order Hold/1 -> LPF vq7/1, To Workspace1/1, [w_abc]

== system Microgrid_24h_Bhutan/Subsystem/Inverter Control  Measurements3/PLL/abc  - d/q ==
  abc : Inport
  tita : Inport  Port=2
  abc  - alfa/beta : Subsystem
  alfa/beta - dq : Subsystem
  d/q : Outport
  wires:
  tita/1 -> alfa/beta - dq/2(tita)
  alfa/beta - dq/1(d/q) -> d/q/1
  abc/1 -> abc  - alfa/beta/1(abc)
  abc  - alfa/beta/1(alfa/beta) -> alfa/beta - dq/1(alfa/beta)

== system Microgrid_24h_Bhutan/Subsystem/Subsystem11/Load Power Calculation1/Subsystem1 ==
  Qacload : Inport
  LPF vq7 : powerlib_extras/Discrete  Control Blocks/Discrete 1st-Order Filter  FilterType=Lowpass  Tc=10e-3  Ts=5e-6  Initialize=off  Vac_Init=[0.8 -25 60]  Vdc_Init=0  PlotResponse=off  param1=[1 100 0.1]
  To Workspace1 : ToWorkspace  VariableName=Qacload3  SampleTime=-1
  To Workspace2 : ToWorkspace  VariableName=Qacload_3  SampleTime=-1
  Zero-Order Hold : ZeroOrderHold  SampleTime=5e-6
  tag scope: Qacload3=global
  wires:
  Qacload/1 -> Zero-Order Hold/1
  Zero-Order Hold/1 -> [Qacload3], To Workspace2/1, LPF vq7/1
  LPF vq7/1 -> To Workspace1/1

== system Microgrid_24h_Bhutan/Subsystem/Subsystem11/Load Power Calculation1/Subsystem2 ==
  Pload : Inport
  LPF vq7 : powerlib_extras/Discrete  Control Blocks/Discrete 1st-Order Filter  FilterType=Lowpass  Tc=10e-3  Ts=5e-6  Initialize=off  Vac_Init=[0.8 -25 60]  Vdc_Init=0  PlotResponse=off  param1=[1 100 0.1]
  To Workspace1 : ToWorkspace  VariableName=Pacload3  SampleTime=-1
  To Workspace2 : ToWorkspace  VariableName=Pacload_3  SampleTime=-1
  Zero-Order Hold : ZeroOrderHold  SampleTime=5e-6
  tag scope: Pacload3=global
  wires:
  Pload/1 -> Zero-Order Hold/1
  Zero-Order Hold/1 -> [Pacload3], To Workspace2/1, LPF vq7/1
  LPF vq7/1 -> To Workspace1/1

== system Microgrid_24h_Bhutan/Subsystem/Subsystem11/Load Power Calculation2/Subsystem1 ==
  Qacload : Inport
  LPF vq7 : powerlib_extras/Discrete  Control Blocks/Discrete 1st-Order Filter  FilterType=Lowpass  Tc=10e-3  Ts=5e-6  Initialize=off  Vac_Init=[0.8 -25 60]  Vdc_Init=0  PlotResponse=off  param1=[1 100 0.1]
  To Workspace1 : ToWorkspace  VariableName=Qacload2  SampleTime=-1
  To Workspace2 : ToWorkspace  VariableName=Qacload_2  SampleTime=-1
  Zero-Order Hold : ZeroOrderHold  SampleTime=5e-6
  tag scope: Qacload2=global
  wires:
  Qacload/1 -> Zero-Order Hold/1
  Zero-Order Hold/1 -> [Qacload2], To Workspace2/1, LPF vq7/1
  LPF vq7/1 -> To Workspace1/1

== system Microgrid_24h_Bhutan/Subsystem/Subsystem11/Load Power Calculation2/Subsystem2 ==
  Pload : Inport
  LPF vq7 : powerlib_extras/Discrete  Control Blocks/Discrete 1st-Order Filter  FilterType=Lowpass  Tc=10e-3  Ts=5e-6  Initialize=off  Vac_Init=[0.8 -25 60]  Vdc_Init=0  PlotResponse=off  param1=[1 100 0.1]
  To Workspace1 : ToWorkspace  VariableName=Pacload2  SampleTime=-1
  To Workspace2 : ToWorkspace  VariableName=Pacload_2  SampleTime=-1
  Zero-Order Hold : ZeroOrderHold  SampleTime=5e-6
  tag scope: Pacload2=global
  wires:
  Pload/1 -> Zero-Order Hold/1
  Zero-Order Hold/1 -> [Pacload2], To Workspace2/1, LPF vq7/1
  LPF vq7/1 -> To Workspace1/1

== system Microgrid_24h_Bhutan/Subsystem/Inverter Control  Measurements3/PLL/abc  - d/q/abc  - alfa/beta ==
  abc : Inport
  Mux : Mux  Inputs=2
  d_s : Fcn  Expr=(-1/sqrt(3)*u[2])+(1/sqrt(3)*u[3])
  q_s : Fcn  Expr=(2/3)*u[1]-(1/3)*u[2]-(1/3)*u[3]
  alfa/beta : Outport
  wires:
  abc/1 -> q_s/1, d_s/1
  d_s/1 -> Mux/1
  q_s/1 -> Mux/2
  Mux/1 -> alfa/beta/1

== system Microgrid_24h_Bhutan/Subsystem/Inverter Control  Measurements3/PLL/abc  - d/q/alfa/beta - dq ==
  alfa/beta : Inport
  tita : Inport  Port=2
  Mux : Mux  Inputs=2
  Mux1 : Mux  Inputs=2
  d : Fcn  Expr=u[2]*sin(u[3]) + u[1]*cos(u[3])
  q : Fcn  Expr=-u[1]*sin(u[3]) + u[2]*cos(u[3])
  d/q : Outport
  wires:
  d/1 -> Mux/1
  q/1 -> Mux/2
  Mux/1 -> d/q/1
  alfa/beta/1 -> Mux1/1
  tita/1 -> Mux1/2
  Mux1/1 -> d/1, q/1

== matlab function PV Array/PV ==
  data: Vpv input double; Ipv output double; Irr input double; TaC input double
function Ipv = Photovoltaic(Vpv,Irr,TaC)

%% REFERENCE PAPER:
% Francisco M. González-Longatt, "Model of Photovoltaic Module inMatlabTM",
% II CIBELEC 2005.

%% Solar panel: Suntech STP-280S
% photovoltaic.m function calculates solar array current with a 
% given voltage, irradiance and temperature
% Ipv = photovoltaic array current (function output)
% Vpv = photovoltaic array voltage
% Irr = irradiance (1 Irr = 1000 W/m^2)
% TaC = temperature (in celsius degrees)

%% Constants

k = 1.38e-23;        % Boltzman’s const
q = 1.60e-19;        % charge on an electron
Np = 10;             % Number of solar panels
n = 2;               % Diode quality factor (=2 for crystaline, <2 for amorphous)
Vg = 1.12;           % Band gap voltage, 1.12V for xtal Si, 1.75 for amorphous Si
Ns = 72*Np;          % Number of cells conected in series (96 cells each panel) 96
T1 = 273 + 25;       % 25C degrees in Kelvin's
Voc_T1 = 44.8*Np/Ns; % Open circuit voltage per cell at T1 temperature 64.2
Isc_T1 = 8.33;       % Short circuit current at temperature T1 5.96

T2 = 273 + 75;
Voc_T2 = Voc_T1*(-0.34/100*(T2-T1)) /Ns; % Open circuit voltage per cell at temperature T2
Isc_T2 = Isc_T1*(0.05/100*(T2-T1));      % Short circuit current per cell at temperature T2

TaK = 273 + TaC; % Photovoltaic array working temperature
TrK = 273 + 25;  % Reference temperature

%% Calculation of the photocurrent Iph
K0 = (Isc_T2 - Isc_T1)/(T2-T1);          % K0 constant is determined from Isc vs T (ECUATION 4)
Iph_T1 = Isc_T1 * Irr;                   % (ECUATION 3)
Iph = Iph_T1 + K0*(TaK-T1);              % Photocurrent (ECUATION 2)

%% Calculation of saturation current of the diode I0
I0_T1 = Isc_T1/(exp(q*Voc_T1/(n*k*T1))-1);                       % (ECUATION 6)
I0 = I0_T1*(TaK/T1).^(3/n).*exp(-q*Vg/(n*k).*((1./TaK)-(1/T1))); % Diode sat. current

%% Calculation of the series resistance Rs, represents the resistance inside
%  its cell in the connection between cells
Xv = I0_T1*q/(n*k*T1)*exp(q*Voc_T1/(n*k*T1)); % (ECUATION 8)
dVdI_Voc = -1.15/Ns /2;                       % dV/dI at Vco per cell, from manufacturers graph
Rs = -dVdI_Voc - 1/Xv;                        % Resistance per cell (ECUATION 7)

%% Calculation of the PV array current, Ipv
Vt_Ta = n*k*TaK/q;                            % = nkT/q
Vc = Vpv/Ns;
Ipv = zeros(size(Vc));
% Ipv = Iph - I0.*( exp((Vc+Ipv.*Rs)./Vt_Ta) -1) (ECUATION 1);
% Solve for Ipv: f(Ipv) = Iph - Ipv - I0.*( exp((Vc+Ia.*Rs)./Vt_Ta) -1) = 0;
% Newton-Raphson method: Ipv2 = Ipv1 - f(Ipv1)/f’(Ipv1)
for j=1:5;
  Ipv = Ipv - ...
  (Iph - Ipv - I0.*( exp((Vc+Ipv.*Rs)./Vt_Ta) -1))...
  ./ (-1 - (I0.*( exp((Vc+Ipv.*Rs)./Vt_Ta) -1)).*Rs./Vt_Ta);
end

== matlab function Boost/Incremental Conductance MPPT/MPPT IC ==
  data: delta output double; Ipv input double; Iprevious input double; Vref output double; Vpv input double; Vprevious input double; Vref_previous input double; Ipv_prev_out output double; Vpv_prev_out output double
function [delta,Vref,Ipv_prev_out,Vpv_prev_out] = IncCond(Ipv,Iprevious,Vpv,Vprevious,Vref_previous)

% REFERENCE PAPERS:
% Trishan Esram, Patrick L. Chapman, "Comparison of Photovoltaic Array
% Maximum Power Tracking Techniques", IEEE Transactions on Energy
% COnversion, vol. 22, issue 2, June 2007.
%
% M. Lokanadham, K. Vijaya Bhaskar, "Incremental Conductance Based Maximum
% Power Point Tracking (MPPT) for Photovoltaic System" International
% Journal of Engineering Research and Applications (IJERA), vol. 2, issue
% 2, March-April 2012.


% The followoing code is an algorithm for a Maximum Power Point Tracking
% (MPPT) technique Incremental COnductance

Vbus = 600;

dI=Ipv-Iprevious;
dV=Vpv-Vprevious;

if (dV==0)
    if (dI==0)
        Vref=Vref_previous;
    else
        if (Ipv>0)
            Vref= Vpv+dV;
        else
            Vref= Vpv-dV;
        end
    end
else
    if ((dI/dV)==(-Ipv/Vpv))
        Vref=Vref_previous;
    else
        if ((dI/dV)>(-Ipv/Vpv))
            Vref= Vpv+dV;
        else
            Vref= Vpv-dV;
        end
    end
end
Ipv_prev_out=Ipv;
Vpv_prev_out=Vpv;

delta=1-Vref/Vbus;

end
